simulink model "ssc_lithium_battery_80Cells"  (Simulink 7.6)
settings: Solver=ode15s  StartTime=0.0  StopTime=40000  MaxStep=600  RelTol=1e-3
PreLoadFcn:
  | ssc_lithium_battery_80Cells_ini
values from neighbouring files (symbols this model uses):
  BatteryParams = struct()    [ssc_lithium_battery_80Cells_ini.m]
undefined symbols (not defined in the file or in its folder): sigbuilder_block
libraries: fl_lib x26, LiBatteryBlocks x11, nesl_utility x4
settings Model: Creator=rjackey  LastModifiedBy=rjackey
settings DebuggingCC: FcnCallInpInsideContextMsg=Enable All
settings GRTTargetCC: CombineOutputUpdateFcns=on

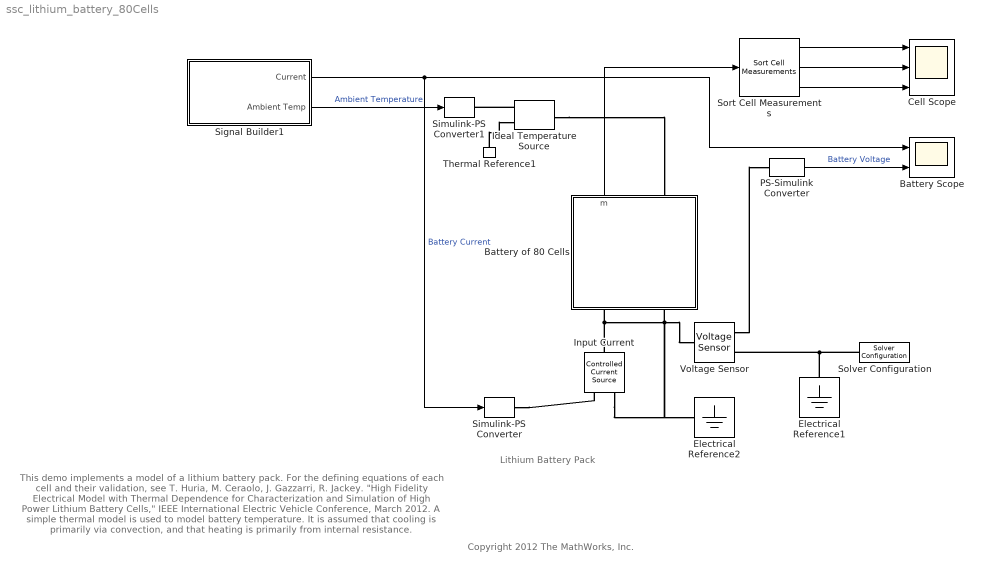
== system ssc_lithium_battery_80Cells ==
  note: Lithium Battery Pack
  note: This demo implements a model of a lithium battery pack. For the defining equations of each cell and their validation, see T. Huria, M. Ceraolo,
      | J. Gazzarri, R. Jackey. "High Fidelity Electrical Model with Thermal Dependence for Characterization and Simulation of High Power Lithium
      | Battery Cells," IEEE International Electric Vehicle Conference, March 2012. A simple thermal model is used to model battery temperature. It is
      | assumed that cooling is primarily via convection, and that heating is primarily from internal resistance.
  note: Copyright 2012 The MathWorks, Inc.
  Battery Scope : Scope  NumInputPorts=2
      settings: TimeRange=40000  YMin=-30~250  YMax=10~340
  Battery of 80 Cells : Subsystem
  Cell Scope : Scope  NumInputPorts=3
      settings: TimeRange=40000  YMin=3~-0.2~20  YMax=4.5~1.2~45
  Electrical Reference1 : fl_lib/Electrical/Electrical Elements/Electrical Reference  DialogController=NetworkEngine.DynNeDlgSource  SystemSampleTime=-1  i_Log=off  LocalVarNames=|i  LocalVarDescs=|i  LocalVarLogging=0
  Electrical Reference2 : fl_lib/Electrical/Electrical Elements/Electrical Reference  DialogController=NetworkEngine.DynNeDlgSource  SystemSampleTime=-1  i_Log=off  LocalVarNames=|i  LocalVarDescs=|i  LocalVarLogging=0
  Ideal Temperature Source : fl_lib/Thermal/Thermal Sources/Ideal Temperature Source  DialogController=NetworkEngine.DynNeDlgSource  SystemSampleTime=-1  Q_Log=off  T_Log=off  LocalVarNames=|heat_flow|T_differential  LocalVarDescs=|Heat flow rate through the source (J/s)|Temperature differential across the source (K)  LocalVarLogging=[0 0]
  Input Current : fl_lib/Electrical/Electrical Sources/Controlled Current Source  DialogController=NetworkEngine.DynNeDlgSource  SystemSampleTime=-1  i_Log=off  v_Log=off  LocalVarNames=|current|voltage|power  LocalVarDescs=|Current (A)|Voltage (V)|Power (W)  LocalVarLogging=[0 0 0]
  PS-Simulink Converter : nesl_utility/PS-Simulink Converter  DialogController=NetworkEngine.DynNeUtilDlgSource  SystemSampleTime=-1  PhysicalDomain=network_engine_domain  LeftPortType=input  RightPortType=output  SubClassName=ps_output  Unit=V  AffineConversion=off
  Signal Builder1 : Subsystem  Tag=STV Subsys  LoadFcn=sigbuilder_block('load');  StartFcn=sigbuilder_block('start');  StopFcn=sigbuilder_block('stop');  ClipboardFcn=sigbuilder_block('clipboard');  mask(Sigbuilder block){}
      mask help: Simulink:masks:SigbuilderBlock_MD
      mask init:
      | if ~strcmp(get_param(bdroot(gcbh),'SimulationStatus'),'stopped') tuvar = sigbuilder_block('maskInit'); end
      settings: CopyFcn=sigbuilder_block('copy');  DeleteFcn=sigbuilder_block('delete');  ModelCloseFcn=sigbuilder_block('modelClose');  PreSaveFcn=sigbuilder_block('preSave');  NameChangeFcn=sigbuilder_block('namechange');  OpenFcn=sigbuilder_block('open',[28.5 123.75 755.25 399.75 ]);  CloseFcn=sigbuilder_block('close');
      mask Display: plot(0,0,100,100,[10,10,40,40,10],[80,20,20,80,80],[40,10],[50,50], [40,27,10],[65,72,56],[40,25,25,10],[28,28,43,43]);
  Simulink-PS Converter : nesl_utility/Simulink-PS Converter  DialogController=NetworkEngine.DynNeUtilDlgSource  SystemSampleTime=-1  PhysicalDomain=network_engine_domain  LeftPortType=input  RightPortType=output  SubClassName=ps_input  Unit=A  AffineConversion=on  InputFilterTimeConstant=.001  UdotUserProvided=0
  Simulink-PS Converter1 : nesl_utility/Simulink-PS Converter  DialogController=NetworkEngine.DynNeUtilDlgSource  SystemSampleTime=-1  PhysicalDomain=network_engine_domain  LeftPortType=input  RightPortType=output  SubClassName=ps_input  Unit=C  AffineConversion=on  InputFilterTimeConstant=.001  UdotUserProvided=0
  Solver Configuration : nesl_utility/Solver Configuration  DialogController=NetworkEngine.DynNeUtilDlgSource  SystemSampleTime=-1  PhysicalDomain=network_engine_domain  LeftPortType=input  RightPortType=generic  SubClassName=solver  Accelerate=off  Profile=off  ResidualTolerance=1e-9  MaxNonlinIter=3  MaxModeIter=2  DoFixedCost=off  UseLocalSampling=off  DoDC=off  LinearAlgebra=Sparse  LocalSolverSampleTime=.001  LocalSolverChoice=NE_BACKWARD_EULER_ADVANCER  UseLocalSolver=off
  Sort Cell Measurements : LiBatteryBlocks/Sort Cell Measurements  SystemSampleTime=-1
  Thermal Reference1 : fl_lib/Thermal/Thermal Elements/Thermal Reference  DialogController=NetworkEngine.DynNeDlgSource  SystemSampleTime=-1  Q_Log=off  LocalVarNames=|Q  LocalVarDescs=|Q  LocalVarLogging=[]
  Voltage Sensor : fl_lib/Electrical/Electrical Sensors/Voltage Sensor  DialogController=NetworkEngine.DynNeDlgSource  SystemSampleTime=-1  i1_Log=off  v1_Log=off  LocalVarNames=|i1|v1  LocalVarDescs=|i1|v1  LocalVarLogging=[0 0]
  wires:
  Sort Cell Measurements/2 -> Cell Scope/2
  Sort Cell Measurements/3 -> Cell Scope/3
  PS-Simulink Converter/1 -> Battery Scope/2  "Battery Voltage"
  Battery of 80 Cells/1(m) -> Sort Cell Measurements/1
  Signal Builder1/1(Current) -> Simulink-PS Converter/1, Battery Scope/1  "Battery Current"
  Signal Builder1/2(Ambient Temp) -> Simulink-PS Converter1/1  "Ambient Temperature"
  Sort Cell Measurements/1 -> Cell Scope/1
  connections:
  Ideal Temperature Source/RConn1 -- Simulink-PS Converter1/RConn1
  Thermal Reference1/LConn1 -- Ideal Temperature Source/RConn2
  Simulink-PS Converter/RConn1 -- Input Current/RConn1
  Electrical Reference1/LConn1 -- Voltage Sensor/RConn2 -- Solver Configuration/RConn1
  Battery of 80 Cells/LConn1 -- Voltage Sensor/LConn1 -- Input Current/LConn1
  Battery of 80 Cells/LConn2 -- Input Current/RConn2 -- Electrical Reference2/LConn1
  Voltage Sensor/RConn1 -- PS-Simulink Converter/LConn1
  Ideal Temperature Source/LConn1 -- Battery of 80 Cells/RConn1

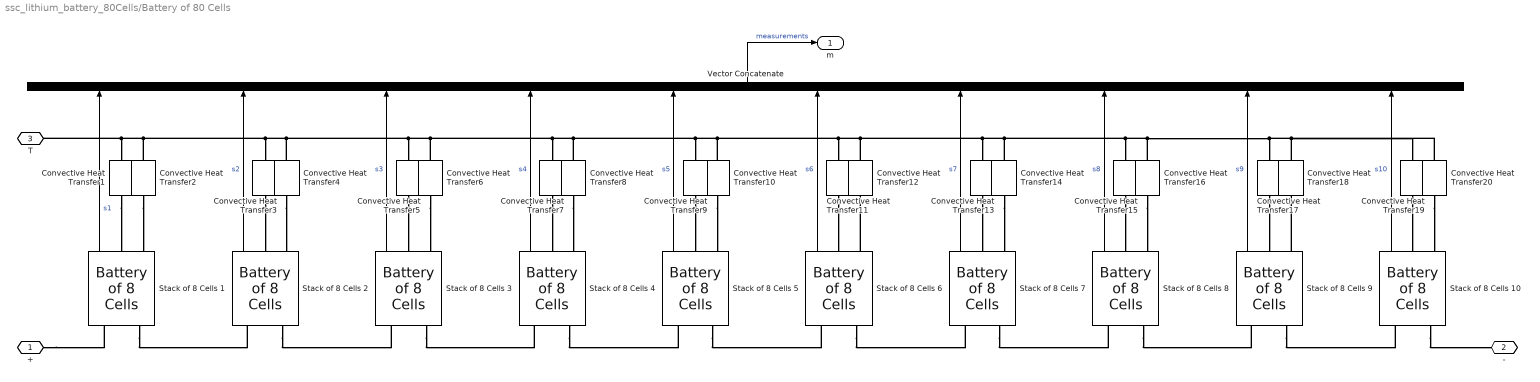
== system ssc_lithium_battery_80Cells/Battery of 80 Cells ==
  Convective Heat Transfer{1..20} (20 alike) : fl_lib/Thermal/Thermal Elements/Convective Heat Transfer  DialogController=NetworkEngine.DynNeDlgSource  SystemSampleTime=-1  area=cell_area m^2  heat_tr_coeff=h_conv_end W/(m^2 * K)  Q_Log=off  T_Log=off  LocalVarNames=|heat_flow|temperature_diff  LocalVarDescs=|Heat flow (J/s)|Temperature difference (K)  LocalVarLogging=[0 0]
  Stack of 8 Cells {1..10} (10 alike) : LiBatteryBlocks/Battery of 8 Cells  SystemSampleTime=-1  ThisStackParams=BatteryParams(1:8)
      settings: AttributesFormatString=%<ThisStackParams>
  Vector Concatenate : Concatenate  NumInputs=10  Mode=Vector
  + : PMIOPort  Port=1  Side=Left
  - : PMIOPort  Port=2  Side=Left
  T : PMIOPort  Port=3  Side=Right
  m : Outport
  wires:
  Vector Concatenate/1 -> m/1  "measurements"
  Stack of 8 Cells 1/1 -> Vector Concatenate/1  "s1"
  Stack of 8 Cells 2/1 -> Vector Concatenate/2  "s2"
  Stack of 8 Cells 3/1 -> Vector Concatenate/3  "s3"
  Stack of 8 Cells 4/1 -> Vector Concatenate/4  "s4"
  Stack of 8 Cells 5/1 -> Vector Concatenate/5  "s5"
  Stack of 8 Cells 6/1 -> Vector Concatenate/6  "s6"
  Stack of 8 Cells 7/1 -> Vector Concatenate/7  "s7"
  Stack of 8 Cells 8/1 -> Vector Concatenate/8  "s8"
  Stack of 8 Cells 9/1 -> Vector Concatenate/9  "s9"
  Stack of 8 Cells 10/1 -> Vector Concatenate/10  "s10"
  connections:
  Convective Heat Transfer16/LConn1 -- Convective Heat Transfer15/LConn1 -- Convective Heat Transfer14/LConn1 -- Convective Heat Transfer13/LConn1 -- Convective Heat Transfer12/LConn1 -- Convective Heat Transfer11/LConn1 -- Convective Heat Transfer10/LConn1 -- Convective Heat Transfer9/LConn1 -- Convective Heat Transfer8/LConn1 -- Convective Heat Transfer7/LConn1 -- Convective Heat Transfer6/LConn1 -- Convective Heat Transfer5/LConn1 -- Convective Heat Transfer4/LConn1 -- Convective Heat Transfer3/LConn1 -- Convective Heat Transfer2/LConn1 -- Convective Heat Transfer1/LConn1 -- T/RConn1 -- Convective Heat Transfer18/LConn1 -- Convective Heat Transfer20/LConn1 -- Convective Heat Transfer19/LConn1 -- Convective Heat Transfer17/LConn1
  +/RConn1 -- Stack of 8 Cells 1/LConn1
  Stack of 8 Cells 1/LConn2 -- Stack of 8 Cells 2/LConn1
  Stack of 8 Cells 3/LConn2 -- Stack of 8 Cells 4/LConn1
  Stack of 8 Cells 2/LConn2 -- Stack of 8 Cells 3/LConn1
  Stack of 8 Cells 5/LConn2 -- Stack of 8 Cells 6/LConn1
  Stack of 8 Cells 4/LConn2 -- Stack of 8 Cells 5/LConn1
  Stack of 8 Cells 7/LConn2 -- Stack of 8 Cells 8/LConn1
  Stack of 8 Cells 6/LConn2 -- Stack of 8 Cells 7/LConn1
  Stack of 8 Cells 8/LConn2 -- Stack of 8 Cells 9/LConn1
  Stack of 8 Cells 9/LConn2 -- Stack of 8 Cells 10/LConn1
  Stack of 8 Cells 10/LConn2 -- -/RConn1
  Convective Heat Transfer1/RConn1 -- Stack of 8 Cells 1/RConn1
  Convective Heat Transfer3/RConn1 -- Stack of 8 Cells 2/RConn1
  Convective Heat Transfer5/RConn1 -- Stack of 8 Cells 3/RConn1
  Convective Heat Transfer7/RConn1 -- Stack of 8 Cells 4/RConn1
  Convective Heat Transfer9/RConn1 -- Stack of 8 Cells 5/RConn1
  Convective Heat Transfer11/RConn1 -- Stack of 8 Cells 6/RConn1
  Convective Heat Transfer13/RConn1 -- Stack of 8 Cells 7/RConn1
  Convective Heat Transfer15/RConn1 -- Stack of 8 Cells 8/RConn1
  Convective Heat Transfer17/RConn1 -- Stack of 8 Cells 9/RConn1
  Convective Heat Transfer19/RConn1 -- Stack of 8 Cells 10/RConn1
  Convective Heat Transfer20/RConn1 -- Stack of 8 Cells 10/RConn2
  Stack of 8 Cells 9/RConn2 -- Convective Heat Transfer18/RConn1
  Convective Heat Transfer16/RConn1 -- Stack of 8 Cells 8/RConn2
  Convective Heat Transfer14/RConn1 -- Stack of 8 Cells 7/RConn2
  Stack of 8 Cells 6/RConn2 -- Convective Heat Transfer12/RConn1
  Convective Heat Transfer10/RConn1 -- Stack of 8 Cells 5/RConn2
  Convective Heat Transfer8/RConn1 -- Stack of 8 Cells 4/RConn2
  Convective Heat Transfer6/RConn1 -- Stack of 8 Cells 3/RConn2
  Convective Heat Transfer4/RConn1 -- Stack of 8 Cells 2/RConn2
  Convective Heat Transfer2/RConn1 -- Stack of 8 Cells 1/RConn2

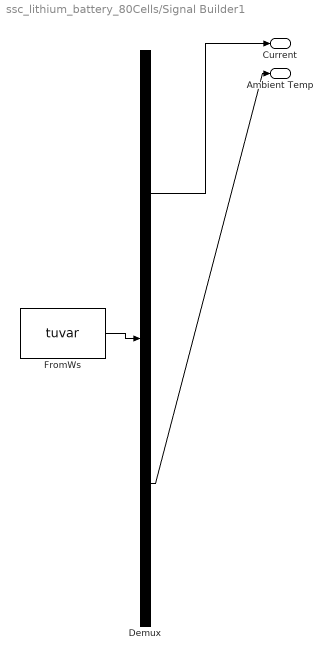
== system ssc_lithium_battery_80Cells/Signal Builder1 ==
  Demux : Demux  Tag=STV Demux  Outputs=2
  FromWs : FromWorkspace  Tag=STV FromWs  VariableName=tuvar  SampleTime=0  SigBuilderData=DataTag0  VnvData=DataTag1
      SigBuilderData=|
      | common.afterFinalStr = 'Extrapolate'
      | common.sampleTime = 0
      | dataSet(1).timeRange = [0 40000]
      | dataSet(1).name = 'Pulse'
      | dataSet(2).timeRange = [0 40000]
      | dataSet(2).name = 'Constant'
      | sbobj.Name = 'Signal Builder'
      | sbobj.Groups(1).Name = 'Pulse'
      | sbobj.Groups(1).Signals(1).Name = 'Current'
      | sbobj.Groups(1).Signals(1).XData = [0 300 300 1900 1900 3600 3600 3960 3960 7200 7200 7560 7560 10800 10800 11160 11160 14400 14400 14760 14760 18000 18000 18360 18360 21600 21600 21960 21960 25200 25200 25560 25560 28800 28800 29160 29160 32400 32400 32760 32760 36000 36000 36360 36360 40000]
      | sbobj.Groups(1).Signals(1).YData = [0 0 7 7 0 0 -27.625 -27.625 0 0 -27.625 -27.625 0 0 -27.625 -27.625 0 0 -27.625 -27.625 0 0 -27.625 -27.625 0 0 -27.625 -27.625 0 0 -27.625 -27.625 0 0 -27.625 -27.625 0 0 -27.625 -27.625 0 0 -27.625 -27.625 0 0]
      | sbobj.Groups(1).Signals(2).Name = 'Ambient Temp'
      | sbobj.Groups(1).Signals(2).XData = [0 300 2100 3600 3960 7200 7560 10800 11160 14400 14760 18000 18360 21600 21960 25200 25560 28800 29160 32400 32760 36000 36360 40000]
      | sbobj.Groups(1).Signals(2).YData = [20 20 20 20 20 20 20 20 20 20 20 20 20 20 20 20 20 20 20 20 20 20 20 20]
      | sbobj.Groups(1).TimeRange = [0 40000]
      | sbobj.Groups(2).Name = 'Constant'
      | sbobj.Groups(2).Signals(1).Name = 'Current'
      | sbobj.Groups(2).Signals(1).XData = [0 360 360 9100 9100 11800 11800 28200 33800 40000]
      | sbobj.Groups(2).Signals(1).YData = [0 0 -5 -5 0 0 5 5 0 0]
      | sbobj.Groups(2).Signals(2).Name = 'Ambient Temp'
      | sbobj.Groups(2).Signals(2).XData = [0 360 360 9100 9100 11800 11800 28200 33800 40000]
      | sbobj.Groups(2).Signals(2).YData = [20 20.09 20.09 22.275 22.275 22.95 22.95 27.05 28.45 30]
      | sbobj.Groups(2).TimeRange = [0 40000]
  Current : Outport
  Ambient Temp : Outport  Tag=STV Outport  Port=2
  wires:
  Demux/1 -> Current/1
  FromWs/1 -> Demux/1
  Demux/2 -> Ambient Temp/1
